simulink model "crc_calculation"  (R2023a)
settings: Solver=VariableStepAuto  StartTime=0.0  StopTime=100e-6  RelTol=1e-3
libraries: simulink x4, hdlsllib x2, simulink_extras x1
settings Model: Creator=micha  LastModifiedBy=micha

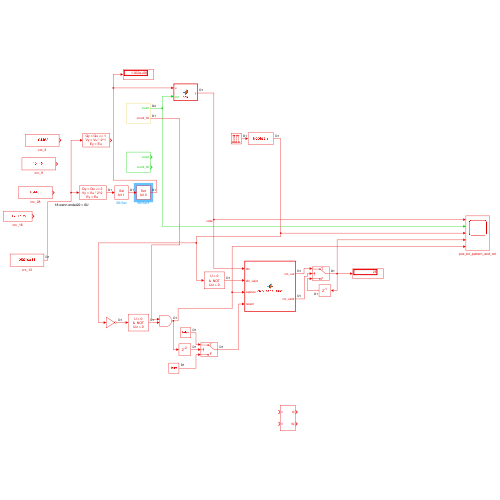
[thumbnail: Simulink's stored preview of the top-level diagram]
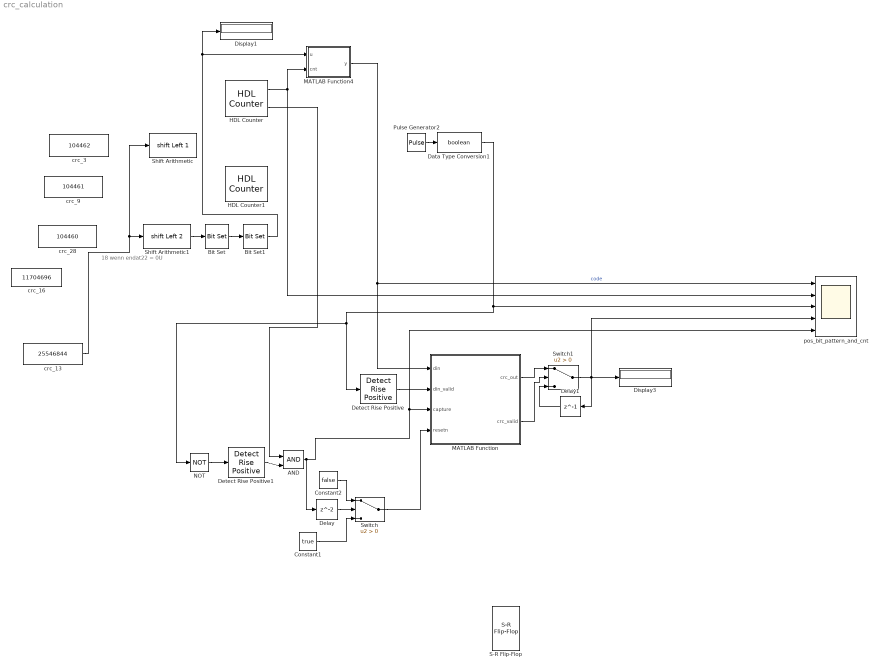
== system crc_calculation ==
  note: 18 wenn endat22 = 0U
  AND : Logic  IconShape=distinctive  AllPortsSameDT=off  OutDataTypeStr=boolean
  Bit Set : simulink/Logic and Bit Operations/Bit Set  iBit=1
  Bit Set1 : simulink/Logic and Bit Operations/Bit Set  iBit=0
  Constant1 : Constant  Value=true  SampleTime=-1
  Constant2 : Constant  Value=false  SampleTime=-1
  Data Type Conversion1 : DataTypeConversion  OutDataTypeStr=boolean  SaturateOnIntegerOverflow=off  RndMeth=Floor
  Delay : Delay
  Delay1 : Delay  DelayLength=1
  Detect Rise Positive : simulink/Logic and Bit Operations/Detect Rise Positive  vinit=0  OutDataTypeStr=boolean
  Detect Rise Positive1 : simulink/Logic and Bit Operations/Detect Rise Positive  vinit=0  OutDataTypeStr=boolean
  Display1 : Display
  Display3 : Display
  HDL Counter : hdlsllib/Sources/HDL Counter  CountType=Count limited  CountInit=1  CountStep=1  CountMax=27  CountFromType=Initial value  CountFrom=1  CountResetPort=off  CountLoadPort=off  CountEnbPort=off  CountDirPort=off  CountHitOutputPort=on  CountDataType=Unsigned  CountWordLen=8  CountFracLen=0  CountSampTime=1e-6
  HDL Counter1 : hdlsllib/Sources/HDL Counter  CountType=Count limited  CountInit=1  CountStep=1  CountMax=26  CountFromType=Initial value  CountFrom=1  CountResetPort=off  CountLoadPort=off  CountEnbPort=off  CountDirPort=off  CountHitOutputPort=on  CountDataType=Unsigned  CountWordLen=8  CountFracLen=0  CountSampTime=1e-6
  MATLAB Function : MATLAB Function  TreatAsAtomicUnit=on
  MATLAB Function4 : MATLAB Function  TreatAsAtomicUnit=on
  NOT : Logic  Operator=NOT  IconShape=distinctive  AllPortsSameDT=off  OutDataTypeStr=boolean
  Pulse Generator2 : DiscretePulseGenerator  Period=10  PulseWidth=5  PhaseDelay=1  SampleTime=0.1e-6
  S-R Flip-Flop : simulink_extras/Flip Flops/S-R Flip-Flop  initial_condition=0
  Shift Arithmetic : ArithShift  BitShiftNumber=1  BitShiftDirection=Left
  Shift Arithmetic1 : ArithShift  BitShiftNumber=2  BitShiftDirection=Left
  Switch : Switch  Criteria=u2 > Threshold  SaturateOnIntegerOverflow=off  InputSameDT=off
  Switch1 : Switch  Criteria=u2 > Threshold  SaturateOnIntegerOverflow=off  InputSameDT=off
  crc_13 : Constant  Value=25546844  OutDataTypeStr=uint32  SampleTime=-1
  crc_16 : Constant  Value=11704696  OutDataTypeStr=uint32  SampleTime=-1
  crc_28 : Constant  Value=104460  OutDataTypeStr=uint32  SampleTime=-1
  crc_3 : Constant  Value=104462  OutDataTypeStr=uint32  SampleTime=-1
  crc_9 : Constant  Value=104461  OutDataTypeStr=uint32  SampleTime=-1
  pos_bit_pattern_and_cnt : Scope  NumInputPorts=5
  wires:
  HDL Counter/1 -> pos_bit_pattern_and_cnt/2, MATLAB Function4/2(cnt)
  MATLAB Function4/1(y) -> MATLAB Function/1(din), pos_bit_pattern_and_cnt/1  "code"
  Bit Set1/1 -> Display1/1, MATLAB Function4/1(u)
  Pulse Generator2/1 -> Data Type Conversion1/1
  Data Type Conversion1/1 -> NOT/1, Detect Rise Positive/1, pos_bit_pattern_and_cnt/3
  crc_13/1 -> Shift Arithmetic/1, Shift Arithmetic1/1
  Detect Rise Positive/1 -> MATLAB Function/2(din_valid)
  HDL Counter/2 -> AND/1
  Switch1/1 -> Delay1/1, Display3/1, pos_bit_pattern_and_cnt/4
  AND/1 -> Delay/1, pos_bit_pattern_and_cnt/5, MATLAB Function/3(capture)
  Detect Rise Positive1/1 -> AND/2
  NOT/1 -> Detect Rise Positive1/1
  Delay/1 -> Switch/2
  Constant1/1 -> Switch/3
  Constant2/1 -> Switch/1
  Switch/1 -> MATLAB Function/4(resetn)
  Delay1/1 -> Switch1/3
  MATLAB Function/1(crc_out) -> Switch1/1
  MATLAB Function/2(crc_valid) -> Switch1/2
  Shift Arithmetic1/1 -> Bit Set/1
  Bit Set/1 -> Bit Set1/1

== matlab function crc_calculation/MATLAB Function ==
  data: din input; crc_out output; din_valid input; capture input; resetn input; crc_valid output
function [crc_out, crc_valid] = crc5_serial_func(din, din_valid, capture, resetn)
%#codegen
% HDL-synthesizable MATLAB Function for 5-bit serial CRC
%
% Inputs:
%   din       : boolean or uint8(0/1) – serial bit
%   din_valid : boolean – update enable
%   capture   : boolean – snapshot inverted CRC
%   resetn    : boolean – active-low synchronous reset
%
% Outputs:
%   crc_out   : uint8 scalar containing CRC in bits [4:0]
%   crc_valid : boolean – pulse when crc_out is updated

    % Persistent CRC flip-flops (state) – matches Verilog ff[4:0]
    persistent ff0 ff1 ff2 ff3 ff4 initialized

    % Persistent initialization on first call
    if isempty(ff0)
        ff0 = true;  % initial state = 1
        ff1 = true;
        ff2 = true;
        ff3 = true;
        ff4 = true;
    end

    % Default output values
    crc_out   = uint8(0);
    crc_valid = false;

    % Handle synchronous active-low reset
    if ~resetn
        ff0 = true;
        ff1 = true;
        ff2 = true;
        ff3 = true;
        ff4 = true;
        return;
    end

    % Convert din to logical
    d = (din ~= 0);

    % Update LFSR when din_valid is asserted
    if din_valid
        % ex = ff[4] XOR din
        ex = xor(ff4, d);

        % next state (matches exactly Verilog/C logic)
        ff0_next = ex;
        ff1_next = xor(ff0, ex);
        ff2_next = ff1;
        ff3_next = xor(ff2, ex);
        ff4_next = ff3;

        % Commit state
        ff0 = ff0_next;
        ff1 = ff1_next;
        ff2 = ff2_next;
        ff3 = ff3_next;
        ff4 = ff4_next;
    end

    % Capture inverted CRC
    if capture
        % Build 5-bit CRC as uint8:
        % order: [ff4 ff3 ff2 ff1 ff0], each inverted, MSB first
        b4 = uint8(~ff4);
        b3 = uint8(~ff3);
        b2 = uint8(~ff2);
        b1 = uint8(~ff1);
        b0 = uint8(~ff0);

        crc_out = bitor( ...
                    bitor( ...
                        bitor( ...
                            bitor(bitshift(b4, 4), bitshift(b3, 3)), ...
                                  bitshift(b2, 2)), ...
                            bitshift(b1, 1)), ...
                    b0 );

        crc_valid = true;
    end
end

== matlab function crc_calculation/MATLAB Function4 ==
  data: u input; y output; cnt input
function y = fcn(u,cnt)
%#codegen
tmp = bitget(u,cnt);
y = tmp;
